simulink model "sedemo_shared_buffer_mgmt"  (Simulink 7.5)
settings: Solver=VariableStepDiscrete  StartTime=0.0  StopTime=10  MaxStep=inf  RelTol=1e-3
undefined symbols (not defined in the file or in its folder): des_subsystemblock, des_subsysteminport, des_subsystemoutport, des_subsystemsupportblock
libraries: simeventstranslate1 x25, simeventssink1 x23, simeventsrouting1 x9, simeventsgates1 x6, simeventsattributes2 x6, simeventsgenerators1 x6, simeventsserver1 x3, simeventsqueue1 x2, simulink x1, simeventsinfo x1
(part 3 of 4)

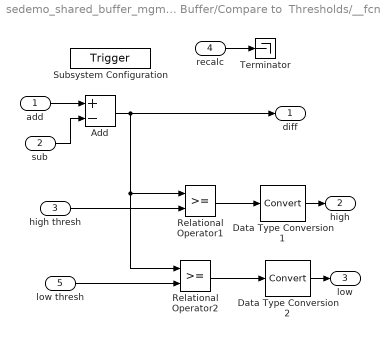
== system sedemo_shared_buffer_mgmt/Receive Buffer/Compare to  Thresholds/__fcn_ss__ ==
  add : Inport  LoadFcn=des_subsysteminport(gcb, 'load');  InitFcn=des_subsysteminport(gcb, 'init');  StartFcn=des_subsysteminport(gcb, 'start');  StopFcn=des_subsysteminport(gcb, 'stop');  OutDataType=sfix(16)  OutScaling=2^0  mask(Discrete Event Inport){PermitSubsystemEvents=on, TypeOfEvent=Change in signal, SignalEdgeOption=Either, SpecifyEventPriority=off, PrioritySubsystemEvent=20}
      mask prompts: PermitSubsystemEvents "Execute subsystem upon signal-based events"; TypeOfEvent "Type of signal-based event:"; SignalEdgeOption "Type of change in signal value:"; SpecifyEventPriority "Resolve simultaneous signal updates according to event priority"; PrioritySubsystemEvent "Event priority:"
      mask help: Input port for a Discrete Event Subsystem block. This block can conditionally execute the subsystem upon signal-based events that meet specified criteria.
      mask init:
      | des_subsystemmask(gcb, 'init','apply')
      settings: CopyFcn=des_subsysteminport(gcb, 'copy');  DeleteFcn=des_subsysteminport(gcb, 'delete');  UndoDeleteFcn=des_subsysteminport(gcb, 'undodelete');  ModelCloseFcn=des_subsysteminport(gcb, 'modelclose');  PreSaveFcn=des_subsysteminport(gcb, 'presave');  NameChangeFcn=des_subsysteminport(gcb, 'namechange');  ParentCloseFcn=des_subsysteminport(gcb, 'parentclose');
      mask Help: helpview(simeventsbhelp);
      mask StyleString: checkbox,popup(Change in signal|Trigger|Sample time hit),popup(Rising|Falling|Either),checkbox,edit
      mask CallbackString: des_subsystemmask(gcb, 'cbPermitSubsystemEvents', 'noapply');|des_subsystemmask(gcb,'cbTypeOfEvent','noapply');||des_subsystemmask(gcb, 'cbSpecifyEventPriority', 'noapply');|
  sub : Inport  LoadFcn=des_subsysteminport(gcb, 'load');  InitFcn=des_subsysteminport(gcb, 'init');  StartFcn=des_subsysteminport(gcb, 'start');  StopFcn=des_subsysteminport(gcb, 'stop');  Port=2  OutDataType=sfix(16)  OutScaling=2^0  mask(Discrete Event Inport){PermitSubsystemEvents=on, TypeOfEvent=Change in signal, SignalEdgeOption=Either, SpecifyEventPriority=on, PrioritySubsystemEvent=20}
      mask prompts: PermitSubsystemEvents "Execute subsystem upon signal-based events"; TypeOfEvent "Type of signal-based event:"; SignalEdgeOption "Type of change in signal value:"; SpecifyEventPriority "Resolve simultaneous signal updates according to event priority"; PrioritySubsystemEvent "Event priority:"
      mask help: Input port for a Discrete Event Subsystem block. This block can conditionally execute the subsystem upon signal-based events that meet specified criteria.
      mask init:
      | des_subsystemmask(gcb, 'init','apply')
      settings: CopyFcn=des_subsysteminport(gcb, 'copy');  DeleteFcn=des_subsysteminport(gcb, 'delete');  UndoDeleteFcn=des_subsysteminport(gcb, 'undodelete');  ModelCloseFcn=des_subsysteminport(gcb, 'modelclose');  PreSaveFcn=des_subsysteminport(gcb, 'presave');  NameChangeFcn=des_subsysteminport(gcb, 'namechange');  ParentCloseFcn=des_subsysteminport(gcb, 'parentclose');
      mask Help: helpview(simeventsbhelp);
      mask StyleString: checkbox,popup(Change in signal|Trigger|Sample time hit),popup(Rising|Falling|Either),checkbox,edit
      mask CallbackString: des_subsystemmask(gcb, 'cbPermitSubsystemEvents', 'noapply');|des_subsystemmask(gcb,'cbTypeOfEvent','noapply');||des_subsystemmask(gcb, 'cbSpecifyEventPriority', 'noapply');|
  high thresh : Inport  LoadFcn=des_subsysteminport(gcb, 'load');  InitFcn=des_subsysteminport(gcb, 'init');  StartFcn=des_subsysteminport(gcb, 'start');  StopFcn=des_subsysteminport(gcb, 'stop');  Port=3  OutDataType=sfix(16)  OutScaling=2^0  mask(Discrete Event Inport){PermitSubsystemEvents=on, TypeOfEvent=Change in signal, SignalEdgeOption=Either, SpecifyEventPriority=off, PrioritySubsystemEvent=20}
      mask prompts: PermitSubsystemEvents "Execute subsystem upon signal-based events"; TypeOfEvent "Type of signal-based event:"; SignalEdgeOption "Type of change in signal value:"; SpecifyEventPriority "Resolve simultaneous signal updates according to event priority"; PrioritySubsystemEvent "Event priority:"
      mask help: Input port for a Discrete Event Subsystem block. This block can conditionally execute the subsystem upon signal-based events that meet specified criteria.
      mask init:
      | des_subsystemmask(gcb, 'init','apply')
      settings: CopyFcn=des_subsysteminport(gcb, 'copy');  DeleteFcn=des_subsysteminport(gcb, 'delete');  UndoDeleteFcn=des_subsysteminport(gcb, 'undodelete');  ModelCloseFcn=des_subsysteminport(gcb, 'modelclose');  PreSaveFcn=des_subsysteminport(gcb, 'presave');  NameChangeFcn=des_subsysteminport(gcb, 'namechange');  ParentCloseFcn=des_subsysteminport(gcb, 'parentclose');
      mask Help: helpview(simeventsbhelp);
      mask StyleString: checkbox,popup(Change in signal|Trigger|Sample time hit),popup(Rising|Falling|Either),checkbox,edit
      mask CallbackString: des_subsystemmask(gcb, 'cbPermitSubsystemEvents', 'noapply');|des_subsystemmask(gcb,'cbTypeOfEvent','noapply');||des_subsystemmask(gcb, 'cbSpecifyEventPriority', 'noapply');|
  recalc : Inport  LoadFcn=des_subsysteminport(gcb, 'load');  InitFcn=des_subsysteminport(gcb, 'init');  StartFcn=des_subsysteminport(gcb, 'start');  StopFcn=des_subsysteminport(gcb, 'stop');  Port=4  OutDataType=sfix(16)  OutScaling=2^0  mask(Discrete Event Inport){PermitSubsystemEvents=on, TypeOfEvent=Change in signal, SignalEdgeOption=Either, SpecifyEventPriority=off, PrioritySubsystemEvent=20}
      mask prompts: PermitSubsystemEvents "Execute subsystem upon signal-based events"; TypeOfEvent "Type of signal-based event:"; SignalEdgeOption "Type of change in signal value:"; SpecifyEventPriority "Resolve simultaneous signal updates according to event priority"; PrioritySubsystemEvent "Event priority:"
      mask help: Input port for a Discrete Event Subsystem block. This block can conditionally execute the subsystem upon signal-based events that meet specified criteria.
      mask init:
      | des_subsystemmask(gcb, 'init','apply')
      settings: CopyFcn=des_subsysteminport(gcb, 'copy');  DeleteFcn=des_subsysteminport(gcb, 'delete');  UndoDeleteFcn=des_subsysteminport(gcb, 'undodelete');  ModelCloseFcn=des_subsysteminport(gcb, 'modelclose');  PreSaveFcn=des_subsysteminport(gcb, 'presave');  NameChangeFcn=des_subsysteminport(gcb, 'namechange');  ParentCloseFcn=des_subsysteminport(gcb, 'parentclose');
      mask Help: helpview(simeventsbhelp);
      mask StyleString: checkbox,popup(Change in signal|Trigger|Sample time hit),popup(Rising|Falling|Either),checkbox,edit
      mask CallbackString: des_subsystemmask(gcb, 'cbPermitSubsystemEvents', 'noapply');|des_subsystemmask(gcb,'cbTypeOfEvent','noapply');||des_subsystemmask(gcb, 'cbSpecifyEventPriority', 'noapply');|
  low thresh : Inport  LoadFcn=des_subsysteminport(gcb, 'load');  InitFcn=des_subsysteminport(gcb, 'init');  StartFcn=des_subsysteminport(gcb, 'start');  StopFcn=des_subsysteminport(gcb, 'stop');  Port=5  OutDataType=sfix(16)  OutScaling=2^0  mask(Discrete Event Inport){PermitSubsystemEvents=on, TypeOfEvent=Change in signal, SignalEdgeOption=Either, SpecifyEventPriority=off, PrioritySubsystemEvent=20}
      mask prompts: PermitSubsystemEvents "Execute subsystem upon signal-based events"; TypeOfEvent "Type of signal-based event:"; SignalEdgeOption "Type of change in signal value:"; SpecifyEventPriority "Resolve simultaneous signal updates according to event priority"; PrioritySubsystemEvent "Event priority:"
      mask help: Input port for a Discrete Event Subsystem block. This block can conditionally execute the subsystem upon signal-based events that meet specified criteria.
      mask init:
      | des_subsystemmask(gcb, 'init','apply')
      settings: CopyFcn=des_subsysteminport(gcb, 'copy');  DeleteFcn=des_subsysteminport(gcb, 'delete');  UndoDeleteFcn=des_subsysteminport(gcb, 'undodelete');  ModelCloseFcn=des_subsysteminport(gcb, 'modelclose');  PreSaveFcn=des_subsysteminport(gcb, 'presave');  NameChangeFcn=des_subsysteminport(gcb, 'namechange');  ParentCloseFcn=des_subsysteminport(gcb, 'parentclose');
      mask Help: helpview(simeventsbhelp);
      mask StyleString: checkbox,popup(Change in signal|Trigger|Sample time hit),popup(Rising|Falling|Either),checkbox,edit
      mask CallbackString: des_subsystemmask(gcb, 'cbPermitSubsystemEvents', 'noapply');|des_subsystemmask(gcb,'cbTypeOfEvent','noapply');||des_subsystemmask(gcb, 'cbSpecifyEventPriority', 'noapply');|
  Subsystem Configuration : TriggerPort  TriggerType=function-call
      settings: CopyFcn=des_subsystemconfigblock(gcb, 'copy');  DeleteFcn=des_subsystemconfigblock(gcb, 'delete');  UndoDeleteFcn=des_subsystemconfigblock(gcb, 'undodelete');
      mask Type: Subsystem Configuration
      mask Description: Configuration for a Discrete Event Subsystem block. Every discrete event subsystem window must contain exactly one copy of this configuration block. Do not delete this block.
      mask Help: helpview(simeventsbhelp);
      mask Display: disp('Do Not Delete');
  Add : Sum  Inputs=+-  OutDataType=sfix(16)  OutScaling=2^-10
  Data Type Conversion1 : DataTypeConversion  OutDataType=sfix(16)  OutScaling=2^0
  Data Type Conversion2 : DataTypeConversion  OutDataType=sfix(16)  OutScaling=2^0
  Relational Operator1 : RelationalOperator  LogicOutDataTypeMode=boolean  OutDataTypeStr=boolean
  Relational Operator2 : RelationalOperator  LogicOutDataTypeMode=boolean  OutDataTypeStr=boolean
  Terminator : Terminator
  diff : Outport  LoadFcn=des_subsystemoutport(gcb, 'load');  InitFcn=des_subsystemoutport(gcb, 'init');  StartFcn=des_subsystemoutport(gcb, 'start');  StopFcn=des_subsystemoutport(gcb, 'stop');  OutDataType=sfix(16)  OutScaling=2^0  mask(Discrete Event Outport){InitOutput=[]}
      mask prompts: InitOutput "Initial output:"
      mask help: Provide an output port for a Discrete Event Subsystem block.
      settings: CopyFcn=des_subsystemoutport(gcb, 'copy');  DeleteFcn=des_subsystemoutport(gcb, 'delete');  UndoDeleteFcn=des_subsystemoutport(gcb, 'undodelete');  ModelCloseFcn=des_subsystemoutport(gcb, 'modelclose');  PreSaveFcn=des_subsystemoutport(gcb, 'presave');  NameChangeFcn=des_subsystemoutport(gcb, 'namechange');  ParentCloseFcn=des_subsystemoutport(gcb, 'parentclose');
      mask Help: helpview(simeventsbhelp);
      mask CallbackString: set_param(gcb,'InitialOutput',get_param(gcb,'InitOutput'));
  high : Outport  LoadFcn=des_subsystemoutport(gcb, 'load');  InitFcn=des_subsystemoutport(gcb, 'init');  StartFcn=des_subsystemoutport(gcb, 'start');  StopFcn=des_subsystemoutport(gcb, 'stop');  Port=2  OutDataType=sfix(16)  OutScaling=2^0  mask(Discrete Event Outport){InitOutput=[]}
      mask prompts: InitOutput "Initial output:"
      mask help: Provide an output port for a Discrete Event Subsystem block.
      settings: CopyFcn=des_subsystemoutport(gcb, 'copy');  DeleteFcn=des_subsystemoutport(gcb, 'delete');  UndoDeleteFcn=des_subsystemoutport(gcb, 'undodelete');  ModelCloseFcn=des_subsystemoutport(gcb, 'modelclose');  PreSaveFcn=des_subsystemoutport(gcb, 'presave');  NameChangeFcn=des_subsystemoutport(gcb, 'namechange');  ParentCloseFcn=des_subsystemoutport(gcb, 'parentclose');
      mask Help: helpview(simeventsbhelp);
      mask CallbackString: set_param(gcb,'InitialOutput',get_param(gcb,'InitOutput'));
  low : Outport  LoadFcn=des_subsystemoutport(gcb, 'load');  InitFcn=des_subsystemoutport(gcb, 'init');  StartFcn=des_subsystemoutport(gcb, 'start');  StopFcn=des_subsystemoutport(gcb, 'stop');  Port=3  OutDataType=sfix(16)  OutScaling=2^0  mask(Discrete Event Outport){InitOutput=[]}
      mask prompts: InitOutput "Initial output:"
      mask help: Provide an output port for a Discrete Event Subsystem block.
      settings: CopyFcn=des_subsystemoutport(gcb, 'copy');  DeleteFcn=des_subsystemoutport(gcb, 'delete');  UndoDeleteFcn=des_subsystemoutport(gcb, 'undodelete');  ModelCloseFcn=des_subsystemoutport(gcb, 'modelclose');  PreSaveFcn=des_subsystemoutport(gcb, 'presave');  NameChangeFcn=des_subsystemoutport(gcb, 'namechange');  ParentCloseFcn=des_subsystemoutport(gcb, 'parentclose');
      mask Help: helpview(simeventsbhelp);
      mask CallbackString: set_param(gcb,'InitialOutput',get_param(gcb,'InitOutput'));
  wires:
  high thresh/1 -> Relational Operator1/2
  add/1 -> Add/1
  sub/1 -> Add/2
  Add/1 -> diff/1, Relational Operator1/1, Relational Operator2/1
  recalc/1 -> Terminator/1
  Data Type Conversion1/1 -> high/1
  Relational Operator1/1 -> Data Type Conversion1/1
  Data Type Conversion2/1 -> low/1
  Relational Operator2/1 -> Data Type Conversion2/1
  low thresh/1 -> Relational Operator2/2

== system sedemo_shared_buffer_mgmt/Receive Buffer/Space Allocated/AAA___ ==

== system sedemo_shared_buffer_mgmt/Receive Buffer/Space Allocated/__fcn_ss__ ==
  add : Inport  LoadFcn=des_subsysteminport(gcb, 'load');  InitFcn=des_subsysteminport(gcb, 'init');  StartFcn=des_subsysteminport(gcb, 'start');  StopFcn=des_subsysteminport(gcb, 'stop');  OutDataType=sfix(16)  OutScaling=2^0  mask(Discrete Event Inport){PermitSubsystemEvents=on, TypeOfEvent=Sample time hit, SignalEdgeOption=Either, SpecifyEventPriority=off, PrioritySubsystemEvent=20}
      mask prompts: PermitSubsystemEvents "Execute subsystem upon signal-based events"; TypeOfEvent "Type of signal-based event:"; SignalEdgeOption "Type of change in signal value:"; SpecifyEventPriority "Resolve simultaneous signal updates according to event priority"; PrioritySubsystemEvent "Event priority:"
      mask help: Input port for a Discrete Event Subsystem block. This block can conditionally execute the subsystem upon signal-based events that meet specified criteria.
      mask init:
      | des_subsystemmask(gcb, 'init','apply')
      settings: CopyFcn=des_subsysteminport(gcb, 'copy');  DeleteFcn=des_subsysteminport(gcb, 'delete');  UndoDeleteFcn=des_subsysteminport(gcb, 'undodelete');  ModelCloseFcn=des_subsysteminport(gcb, 'modelclose');  PreSaveFcn=des_subsysteminport(gcb, 'presave');  NameChangeFcn=des_subsysteminport(gcb, 'namechange');  ParentCloseFcn=des_subsysteminport(gcb, 'parentclose');
      mask Help: helpview(simeventsbhelp);
      mask StyleString: checkbox,popup(Change in signal|Trigger|Sample time hit),popup(Rising|Falling|Either),checkbox,edit
      mask CallbackString: des_subsystemmask(gcb, 'cbPermitSubsystemEvents', 'noapply');|des_subsystemmask(gcb,'cbTypeOfEvent','noapply');||des_subsystemmask(gcb, 'cbSpecifyEventPriority', 'noapply');|
  Subsystem Configuration : TriggerPort  TriggerType=function-call
      settings: CopyFcn=des_subsystemconfigblock(gcb, 'copy');  DeleteFcn=des_subsystemconfigblock(gcb, 'delete');  UndoDeleteFcn=des_subsystemconfigblock(gcb, 'undodelete');
      mask Type: Subsystem Configuration
      mask Description: Configuration for a Discrete Event Subsystem block. Every discrete event subsystem window must contain exactly one copy of this configuration block. Do not delete this block.
      mask Help: helpview(simeventsbhelp);
      mask Display: disp('Do Not Delete');
  Add : Sum  OutDataType=sfix(16)  OutScaling=2^-10
  Unit Delay : UnitDelay  SampleTime=-1
  Acc : Outport  LoadFcn=des_subsystemoutport(gcb, 'load');  InitFcn=des_subsystemoutport(gcb, 'init');  StartFcn=des_subsystemoutport(gcb, 'start');  StopFcn=des_subsystemoutport(gcb, 'stop');  OutDataType=sfix(16)  OutScaling=2^0  mask(Discrete Event Outport){InitOutput=[]}
      mask prompts: InitOutput "Initial output:"
      mask help: Provide an output port for a Discrete Event Subsystem block.
      settings: CopyFcn=des_subsystemoutport(gcb, 'copy');  DeleteFcn=des_subsystemoutport(gcb, 'delete');  UndoDeleteFcn=des_subsystemoutport(gcb, 'undodelete');  ModelCloseFcn=des_subsystemoutport(gcb, 'modelclose');  PreSaveFcn=des_subsystemoutport(gcb, 'presave');  NameChangeFcn=des_subsystemoutport(gcb, 'namechange');  ParentCloseFcn=des_subsystemoutport(gcb, 'parentclose');
      mask Help: helpview(simeventsbhelp);
      mask CallbackString: set_param(gcb,'InitialOutput',get_param(gcb,'InitOutput'));
  wires:
  add/1 -> Add/1
  Unit Delay/1 -> Add/2
  Add/1 -> Unit Delay/1, Acc/1

== system sedemo_shared_buffer_mgmt/Receive Buffer/Space Freed/AAA___ ==

== system sedemo_shared_buffer_mgmt/Receive Buffer/Space Freed/__fcn_ss__ ==
  add : Inport  LoadFcn=des_subsysteminport(gcb, 'load');  InitFcn=des_subsysteminport(gcb, 'init');  StartFcn=des_subsysteminport(gcb, 'start');  StopFcn=des_subsysteminport(gcb, 'stop');  OutDataType=sfix(16)  OutScaling=2^0  mask(Discrete Event Inport){PermitSubsystemEvents=on, TypeOfEvent=Sample time hit, SignalEdgeOption=Either, SpecifyEventPriority=off, PrioritySubsystemEvent=20}
      mask prompts: PermitSubsystemEvents "Execute subsystem upon signal-based events"; TypeOfEvent "Type of signal-based event:"; SignalEdgeOption "Type of change in signal value:"; SpecifyEventPriority "Resolve simultaneous signal updates according to event priority"; PrioritySubsystemEvent "Event priority:"
      mask help: Input port for a Discrete Event Subsystem block. This block can conditionally execute the subsystem upon signal-based events that meet specified criteria.
      mask init:
      | des_subsystemmask(gcb, 'init','apply')
      settings: CopyFcn=des_subsysteminport(gcb, 'copy');  DeleteFcn=des_subsysteminport(gcb, 'delete');  UndoDeleteFcn=des_subsysteminport(gcb, 'undodelete');  ModelCloseFcn=des_subsysteminport(gcb, 'modelclose');  PreSaveFcn=des_subsysteminport(gcb, 'presave');  NameChangeFcn=des_subsysteminport(gcb, 'namechange');  ParentCloseFcn=des_subsysteminport(gcb, 'parentclose');
      mask Help: helpview(simeventsbhelp);
      mask StyleString: checkbox,popup(Change in signal|Trigger|Sample time hit),popup(Rising|Falling|Either),checkbox,edit
      mask CallbackString: des_subsystemmask(gcb, 'cbPermitSubsystemEvents', 'noapply');|des_subsystemmask(gcb,'cbTypeOfEvent','noapply');||des_subsystemmask(gcb, 'cbSpecifyEventPriority', 'noapply');|
  Subsystem Configuration : TriggerPort  TriggerType=function-call
      settings: CopyFcn=des_subsystemconfigblock(gcb, 'copy');  DeleteFcn=des_subsystemconfigblock(gcb, 'delete');  UndoDeleteFcn=des_subsystemconfigblock(gcb, 'undodelete');
      mask Type: Subsystem Configuration
      mask Description: Configuration for a Discrete Event Subsystem block. Every discrete event subsystem window must contain exactly one copy of this configuration block. Do not delete this block.
      mask Help: helpview(simeventsbhelp);
      mask Display: disp('Do Not Delete');
  Add : Sum  OutDataType=sfix(16)  OutScaling=2^-10
  Unit Delay : UnitDelay  SampleTime=-1
  Acc : Outport  LoadFcn=des_subsystemoutport(gcb, 'load');  InitFcn=des_subsystemoutport(gcb, 'init');  StartFcn=des_subsystemoutport(gcb, 'start');  StopFcn=des_subsystemoutport(gcb, 'stop');  OutDataType=sfix(16)  OutScaling=2^0  mask(Discrete Event Outport){InitOutput=[]}
      mask prompts: InitOutput "Initial output:"
      mask help: Provide an output port for a Discrete Event Subsystem block.
      settings: CopyFcn=des_subsystemoutport(gcb, 'copy');  DeleteFcn=des_subsystemoutport(gcb, 'delete');  UndoDeleteFcn=des_subsystemoutport(gcb, 'undodelete');  ModelCloseFcn=des_subsystemoutport(gcb, 'modelclose');  PreSaveFcn=des_subsystemoutport(gcb, 'presave');  NameChangeFcn=des_subsystemoutport(gcb, 'namechange');  ParentCloseFcn=des_subsystemoutport(gcb, 'parentclose');
      mask Help: helpview(simeventsbhelp);
      mask CallbackString: set_param(gcb,'InitialOutput',get_param(gcb,'InitOutput'));
  wires:
  add/1 -> Add/1
  Unit Delay/1 -> Add/2
  Add/1 -> Unit Delay/1, Acc/1

== system sedemo_shared_buffer_mgmt/Rx Priority Throttling/OR/AAA___ ==

== system sedemo_shared_buffer_mgmt/Rx Priority Throttling/OR/__fcn_ss__ ==
  Din : Inport  LoadFcn=des_subsysteminport(gcb, 'load');  InitFcn=des_subsysteminport(gcb, 'init');  StartFcn=des_subsysteminport(gcb, 'start');  StopFcn=des_subsysteminport(gcb, 'stop');  OutDataType=sfix(16)  OutScaling=2^0  mask(Discrete Event Inport){PermitSubsystemEvents=on, TypeOfEvent=Sample time hit, SignalEdgeOption=Rising, SpecifyEventPriority=off, PrioritySubsystemEvent=20}
      mask prompts: PermitSubsystemEvents "Execute subsystem upon signal-based events"; TypeOfEvent "Type of signal-based event:"; SignalEdgeOption "Type of change in signal value:"; SpecifyEventPriority "Resolve simultaneous signal updates according to event priority"; PrioritySubsystemEvent "Event priority:"
      mask help: Input port for a Discrete Event Subsystem block. This block can conditionally execute the subsystem upon signal-based events that meet specified criteria.
      mask init:
      | des_subsystemmask(gcb, 'init','apply')
      settings: CopyFcn=des_subsysteminport(gcb, 'copy');  DeleteFcn=des_subsysteminport(gcb, 'delete');  UndoDeleteFcn=des_subsysteminport(gcb, 'undodelete');  ModelCloseFcn=des_subsysteminport(gcb, 'modelclose');  PreSaveFcn=des_subsysteminport(gcb, 'presave');  NameChangeFcn=des_subsysteminport(gcb, 'namechange');  ParentCloseFcn=des_subsysteminport(gcb, 'parentclose');
      mask Help: helpview(simeventsbhelp);
      mask StyleString: checkbox,popup(Change in signal|Trigger|Sample time hit),popup(Rising|Falling|Either),checkbox,edit
      mask CallbackString: des_subsystemmask(gcb, 'cbPermitSubsystemEvents', 'noapply');|des_subsystemmask(gcb,'cbTypeOfEvent','noapply');||des_subsystemmask(gcb, 'cbSpecifyEventPriority', 'noapply');|
  Din1 : Inport  LoadFcn=des_subsysteminport(gcb, 'load');  InitFcn=des_subsysteminport(gcb, 'init');  StartFcn=des_subsysteminport(gcb, 'start');  StopFcn=des_subsysteminport(gcb, 'stop');  Port=2  OutDataType=sfix(16)  OutScaling=2^0  mask(Discrete Event Inport){PermitSubsystemEvents=on, TypeOfEvent=Sample time hit, SignalEdgeOption=Rising, SpecifyEventPriority=off, PrioritySubsystemEvent=20}
      mask prompts: PermitSubsystemEvents "Execute subsystem upon signal-based events"; TypeOfEvent "Type of signal-based event:"; SignalEdgeOption "Type of change in signal value:"; SpecifyEventPriority "Resolve simultaneous signal updates according to event priority"; PrioritySubsystemEvent "Event priority:"
      mask help: Input port for a Discrete Event Subsystem block. This block can conditionally execute the subsystem upon signal-based events that meet specified criteria.
      mask init:
      | des_subsystemmask(gcb, 'init','apply')
      settings: CopyFcn=des_subsysteminport(gcb, 'copy');  DeleteFcn=des_subsysteminport(gcb, 'delete');  UndoDeleteFcn=des_subsysteminport(gcb, 'undodelete');  ModelCloseFcn=des_subsysteminport(gcb, 'modelclose');  PreSaveFcn=des_subsysteminport(gcb, 'presave');  NameChangeFcn=des_subsysteminport(gcb, 'namechange');  ParentCloseFcn=des_subsysteminport(gcb, 'parentclose');
      mask Help: helpview(simeventsbhelp);
      mask StyleString: checkbox,popup(Change in signal|Trigger|Sample time hit),popup(Rising|Falling|Either),checkbox,edit
      mask CallbackString: des_subsystemmask(gcb, 'cbPermitSubsystemEvents', 'noapply');|des_subsystemmask(gcb,'cbTypeOfEvent','noapply');||des_subsystemmask(gcb, 'cbSpecifyEventPriority', 'noapply');|
  Subsystem Configuration : TriggerPort  TriggerType=function-call
      settings: CopyFcn=des_subsystemconfigblock(gcb, 'copy');  DeleteFcn=des_subsystemconfigblock(gcb, 'delete');  UndoDeleteFcn=des_subsystemconfigblock(gcb, 'undodelete');
      mask Type: Subsystem Configuration
      mask Description: Configuration for a Discrete Event Subsystem block. Every discrete event subsystem window must contain exactly one copy of this configuration block. Do not delete this block.
      mask Help: helpview(simeventsbhelp);
      mask Display: disp('Do Not Delete');
  Logical Operator : Logic  AllPortsSameDT=off  OutDataTypeMode=boolean  OutDataTypeStr=boolean
  Logical Operator1 : Logic  Operator=NOT  AllPortsSameDT=off  OutDataTypeMode=Specify via dialog  LogicDataType=float('double')  OutDataTypeStr=float('double')
  Dout : Outport  LoadFcn=des_subsystemoutport(gcb, 'load');  InitFcn=des_subsystemoutport(gcb, 'init');  StartFcn=des_subsystemoutport(gcb, 'start');  StopFcn=des_subsystemoutport(gcb, 'stop');  OutDataType=sfix(16)  OutScaling=2^0  mask(Discrete Event Outport){InitOutput=[]}
      mask prompts: InitOutput "Initial output:"
      mask help: Provide an output port for a Discrete Event Subsystem block.
      settings: CopyFcn=des_subsystemoutport(gcb, 'copy');  DeleteFcn=des_subsystemoutport(gcb, 'delete');  UndoDeleteFcn=des_subsystemoutport(gcb, 'undodelete');  ModelCloseFcn=des_subsystemoutport(gcb, 'modelclose');  PreSaveFcn=des_subsystemoutport(gcb, 'presave');  NameChangeFcn=des_subsystemoutport(gcb, 'namechange');  ParentCloseFcn=des_subsystemoutport(gcb, 'parentclose');
      mask Help: helpview(simeventsbhelp);
      mask CallbackString: set_param(gcb,'InitialOutput',get_param(gcb,'InitOutput'));
  wires:
  Din/1 -> Logical Operator/1
  Din1/1 -> Logical Operator/2
  Logical Operator/1 -> Logical Operator1/1
  Logical Operator1/1 -> Dout/1

== system sedemo_shared_buffer_mgmt/Rx Priority Throttling/OR1/AAA___ ==

== system sedemo_shared_buffer_mgmt/Rx Priority Throttling/OR1/__fcn_ss__ ==
  Din : Inport  LoadFcn=des_subsysteminport(gcb, 'load');  InitFcn=des_subsysteminport(gcb, 'init');  StartFcn=des_subsysteminport(gcb, 'start');  StopFcn=des_subsysteminport(gcb, 'stop');  OutDataType=sfix(16)  OutScaling=2^0  mask(Discrete Event Inport){PermitSubsystemEvents=on, TypeOfEvent=Sample time hit, SignalEdgeOption=Rising, SpecifyEventPriority=off, PrioritySubsystemEvent=20}
      mask prompts: PermitSubsystemEvents "Execute subsystem upon signal-based events"; TypeOfEvent "Type of signal-based event:"; SignalEdgeOption "Type of change in signal value:"; SpecifyEventPriority "Resolve simultaneous signal updates according to event priority"; PrioritySubsystemEvent "Event priority:"
      mask help: Input port for a Discrete Event Subsystem block. This block can conditionally execute the subsystem upon signal-based events that meet specified criteria.
      mask init:
      | des_subsystemmask(gcb, 'init','apply')
      settings: CopyFcn=des_subsysteminport(gcb, 'copy');  DeleteFcn=des_subsysteminport(gcb, 'delete');  UndoDeleteFcn=des_subsysteminport(gcb, 'undodelete');  ModelCloseFcn=des_subsysteminport(gcb, 'modelclose');  PreSaveFcn=des_subsysteminport(gcb, 'presave');  NameChangeFcn=des_subsysteminport(gcb, 'namechange');  ParentCloseFcn=des_subsysteminport(gcb, 'parentclose');
      mask Help: helpview(simeventsbhelp);
      mask StyleString: checkbox,popup(Change in signal|Trigger|Sample time hit),popup(Rising|Falling|Either),checkbox,edit
      mask CallbackString: des_subsystemmask(gcb, 'cbPermitSubsystemEvents', 'noapply');|des_subsystemmask(gcb,'cbTypeOfEvent','noapply');||des_subsystemmask(gcb, 'cbSpecifyEventPriority', 'noapply');|
  Din1 : Inport  LoadFcn=des_subsysteminport(gcb, 'load');  InitFcn=des_subsysteminport(gcb, 'init');  StartFcn=des_subsysteminport(gcb, 'start');  StopFcn=des_subsysteminport(gcb, 'stop');  Port=2  OutDataType=sfix(16)  OutScaling=2^0  mask(Discrete Event Inport){PermitSubsystemEvents=on, TypeOfEvent=Sample time hit, SignalEdgeOption=Rising, SpecifyEventPriority=off, PrioritySubsystemEvent=20}
      mask prompts: PermitSubsystemEvents "Execute subsystem upon signal-based events"; TypeOfEvent "Type of signal-based event:"; SignalEdgeOption "Type of change in signal value:"; SpecifyEventPriority "Resolve simultaneous signal updates according to event priority"; PrioritySubsystemEvent "Event priority:"
      mask help: Input port for a Discrete Event Subsystem block. This block can conditionally execute the subsystem upon signal-based events that meet specified criteria.
      mask init:
      | des_subsystemmask(gcb, 'init','apply')
      settings: CopyFcn=des_subsysteminport(gcb, 'copy');  DeleteFcn=des_subsysteminport(gcb, 'delete');  UndoDeleteFcn=des_subsysteminport(gcb, 'undodelete');  ModelCloseFcn=des_subsysteminport(gcb, 'modelclose');  PreSaveFcn=des_subsysteminport(gcb, 'presave');  NameChangeFcn=des_subsysteminport(gcb, 'namechange');  ParentCloseFcn=des_subsysteminport(gcb, 'parentclose');
      mask Help: helpview(simeventsbhelp);
      mask StyleString: checkbox,popup(Change in signal|Trigger|Sample time hit),popup(Rising|Falling|Either),checkbox,edit
      mask CallbackString: des_subsystemmask(gcb, 'cbPermitSubsystemEvents', 'noapply');|des_subsystemmask(gcb,'cbTypeOfEvent','noapply');||des_subsystemmask(gcb, 'cbSpecifyEventPriority', 'noapply');|
  Subsystem Configuration : TriggerPort  TriggerType=function-call
      settings: CopyFcn=des_subsystemconfigblock(gcb, 'copy');  DeleteFcn=des_subsystemconfigblock(gcb, 'delete');  UndoDeleteFcn=des_subsystemconfigblock(gcb, 'undodelete');
      mask Type: Subsystem Configuration
      mask Description: Configuration for a Discrete Event Subsystem block. Every discrete event subsystem window must contain exactly one copy of this configuration block. Do not delete this block.
      mask Help: helpview(simeventsbhelp);
      mask Display: disp('Do Not Delete');
  Logical Operator : Logic  AllPortsSameDT=off  OutDataTypeMode=boolean  OutDataTypeStr=boolean
  Logical Operator1 : Logic  Operator=NOT  AllPortsSameDT=off  OutDataTypeMode=Specify via dialog  LogicDataType=float('double')  OutDataTypeStr=float('double')
  Dout : Outport  LoadFcn=des_subsystemoutport(gcb, 'load');  InitFcn=des_subsystemoutport(gcb, 'init');  StartFcn=des_subsystemoutport(gcb, 'start');  StopFcn=des_subsystemoutport(gcb, 'stop');  OutDataType=sfix(16)  OutScaling=2^0  mask(Discrete Event Outport){InitOutput=[]}
      mask prompts: InitOutput "Initial output:"
      mask help: Provide an output port for a Discrete Event Subsystem block.
      settings: CopyFcn=des_subsystemoutport(gcb, 'copy');  DeleteFcn=des_subsystemoutport(gcb, 'delete');  UndoDeleteFcn=des_subsystemoutport(gcb, 'undodelete');  ModelCloseFcn=des_subsystemoutport(gcb, 'modelclose');  PreSaveFcn=des_subsystemoutport(gcb, 'presave');  NameChangeFcn=des_subsystemoutport(gcb, 'namechange');  ParentCloseFcn=des_subsystemoutport(gcb, 'parentclose');
      mask Help: helpview(simeventsbhelp);
      mask CallbackString: set_param(gcb,'InitialOutput',get_param(gcb,'InitOutput'));
  wires:
  Din/1 -> Logical Operator/1
  Din1/1 -> Logical Operator/2
  Logical Operator/1 -> Logical Operator1/1
  Logical Operator1/1 -> Dout/1

== system sedemo_shared_buffer_mgmt/Transmit Buffer/Compare to  Thresholds/AAA___ ==

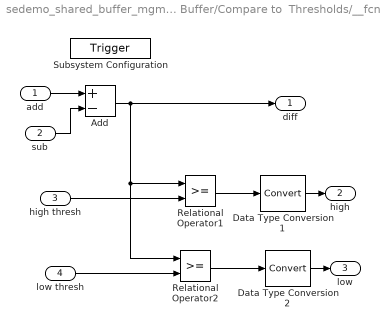
== system sedemo_shared_buffer_mgmt/Transmit Buffer/Compare to  Thresholds/__fcn_ss__ ==
  add : Inport  LoadFcn=des_subsysteminport(gcb, 'load');  InitFcn=des_subsysteminport(gcb, 'init');  StartFcn=des_subsysteminport(gcb, 'start');  StopFcn=des_subsysteminport(gcb, 'stop');  OutDataType=sfix(16)  OutScaling=2^0  mask(Discrete Event Inport){PermitSubsystemEvents=on, TypeOfEvent=Change in signal, SignalEdgeOption=Either, SpecifyEventPriority=off, PrioritySubsystemEvent=20}
      mask prompts: PermitSubsystemEvents "Execute subsystem upon signal-based events"; TypeOfEvent "Type of signal-based event:"; SignalEdgeOption "Type of change in signal value:"; SpecifyEventPriority "Resolve simultaneous signal updates according to event priority"; PrioritySubsystemEvent "Event priority:"
      mask help: Input port for a Discrete Event Subsystem block. This block can conditionally execute the subsystem upon signal-based events that meet specified criteria.
      mask init:
      | des_subsystemmask(gcb, 'init','apply')
      settings: CopyFcn=des_subsysteminport(gcb, 'copy');  DeleteFcn=des_subsysteminport(gcb, 'delete');  UndoDeleteFcn=des_subsysteminport(gcb, 'undodelete');  ModelCloseFcn=des_subsysteminport(gcb, 'modelclose');  PreSaveFcn=des_subsysteminport(gcb, 'presave');  NameChangeFcn=des_subsysteminport(gcb, 'namechange');  ParentCloseFcn=des_subsysteminport(gcb, 'parentclose');
      mask Help: helpview(simeventsbhelp);
      mask StyleString: checkbox,popup(Change in signal|Trigger|Sample time hit),popup(Rising|Falling|Either),checkbox,edit
      mask CallbackString: des_subsystemmask(gcb, 'cbPermitSubsystemEvents', 'noapply');|des_subsystemmask(gcb,'cbTypeOfEvent','noapply');||des_subsystemmask(gcb, 'cbSpecifyEventPriority', 'noapply');|
  sub : Inport  LoadFcn=des_subsysteminport(gcb, 'load');  InitFcn=des_subsysteminport(gcb, 'init');  StartFcn=des_subsysteminport(gcb, 'start');  StopFcn=des_subsysteminport(gcb, 'stop');  Port=2  OutDataType=sfix(16)  OutScaling=2^0  mask(Discrete Event Inport){PermitSubsystemEvents=on, TypeOfEvent=Change in signal, SignalEdgeOption=Either, SpecifyEventPriority=on, PrioritySubsystemEvent=20}
      mask prompts: PermitSubsystemEvents "Execute subsystem upon signal-based events"; TypeOfEvent "Type of signal-based event:"; SignalEdgeOption "Type of change in signal value:"; SpecifyEventPriority "Resolve simultaneous signal updates according to event priority"; PrioritySubsystemEvent "Event priority:"
      mask help: Input port for a Discrete Event Subsystem block. This block can conditionally execute the subsystem upon signal-based events that meet specified criteria.
      mask init:
      | des_subsystemmask(gcb, 'init','apply')
      settings: CopyFcn=des_subsysteminport(gcb, 'copy');  DeleteFcn=des_subsysteminport(gcb, 'delete');  UndoDeleteFcn=des_subsysteminport(gcb, 'undodelete');  ModelCloseFcn=des_subsysteminport(gcb, 'modelclose');  PreSaveFcn=des_subsysteminport(gcb, 'presave');  NameChangeFcn=des_subsysteminport(gcb, 'namechange');  ParentCloseFcn=des_subsysteminport(gcb, 'parentclose');
      mask Help: helpview(simeventsbhelp);
      mask StyleString: checkbox,popup(Change in signal|Trigger|Sample time hit),popup(Rising|Falling|Either),checkbox,edit
      mask CallbackString: des_subsystemmask(gcb, 'cbPermitSubsystemEvents', 'noapply');|des_subsystemmask(gcb,'cbTypeOfEvent','noapply');||des_subsystemmask(gcb, 'cbSpecifyEventPriority', 'noapply');|
  high thresh : Inport  LoadFcn=des_subsysteminport(gcb, 'load');  InitFcn=des_subsysteminport(gcb, 'init');  StartFcn=des_subsysteminport(gcb, 'start');  StopFcn=des_subsysteminport(gcb, 'stop');  Port=3  OutDataType=sfix(16)  OutScaling=2^0  mask(Discrete Event Inport){PermitSubsystemEvents=on, TypeOfEvent=Change in signal, SignalEdgeOption=Either, SpecifyEventPriority=off, PrioritySubsystemEvent=20}
      mask prompts: PermitSubsystemEvents "Execute subsystem upon signal-based events"; TypeOfEvent "Type of signal-based event:"; SignalEdgeOption "Type of change in signal value:"; SpecifyEventPriority "Resolve simultaneous signal updates according to event priority"; PrioritySubsystemEvent "Event priority:"
      mask help: Input port for a Discrete Event Subsystem block. This block can conditionally execute the subsystem upon signal-based events that meet specified criteria.
      mask init:
      | des_subsystemmask(gcb, 'init','apply')
      settings: CopyFcn=des_subsysteminport(gcb, 'copy');  DeleteFcn=des_subsysteminport(gcb, 'delete');  UndoDeleteFcn=des_subsysteminport(gcb, 'undodelete');  ModelCloseFcn=des_subsysteminport(gcb, 'modelclose');  PreSaveFcn=des_subsysteminport(gcb, 'presave');  NameChangeFcn=des_subsysteminport(gcb, 'namechange');  ParentCloseFcn=des_subsysteminport(gcb, 'parentclose');
      mask Help: helpview(simeventsbhelp);
      mask StyleString: checkbox,popup(Change in signal|Trigger|Sample time hit),popup(Rising|Falling|Either),checkbox,edit
      mask CallbackString: des_subsystemmask(gcb, 'cbPermitSubsystemEvents', 'noapply');|des_subsystemmask(gcb,'cbTypeOfEvent','noapply');||des_subsystemmask(gcb, 'cbSpecifyEventPriority', 'noapply');|
  low thresh : Inport  LoadFcn=des_subsysteminport(gcb, 'load');  InitFcn=des_subsysteminport(gcb, 'init');  StartFcn=des_subsysteminport(gcb, 'start');  StopFcn=des_subsysteminport(gcb, 'stop');  Port=4  OutDataType=sfix(16)  OutScaling=2^0  mask(Discrete Event Inport){PermitSubsystemEvents=on, TypeOfEvent=Change in signal, SignalEdgeOption=Either, SpecifyEventPriority=off, PrioritySubsystemEvent=20}
      mask prompts: PermitSubsystemEvents "Execute subsystem upon signal-based events"; TypeOfEvent "Type of signal-based event:"; SignalEdgeOption "Type of change in signal value:"; SpecifyEventPriority "Resolve simultaneous signal updates according to event priority"; PrioritySubsystemEvent "Event priority:"
      mask help: Input port for a Discrete Event Subsystem block. This block can conditionally execute the subsystem upon signal-based events that meet specified criteria.
      mask init:
      | des_subsystemmask(gcb, 'init','apply')
      settings: CopyFcn=des_subsysteminport(gcb, 'copy');  DeleteFcn=des_subsysteminport(gcb, 'delete');  UndoDeleteFcn=des_subsysteminport(gcb, 'undodelete');  ModelCloseFcn=des_subsysteminport(gcb, 'modelclose');  PreSaveFcn=des_subsysteminport(gcb, 'presave');  NameChangeFcn=des_subsysteminport(gcb, 'namechange');  ParentCloseFcn=des_subsysteminport(gcb, 'parentclose');
      mask Help: helpview(simeventsbhelp);
      mask StyleString: checkbox,popup(Change in signal|Trigger|Sample time hit),popup(Rising|Falling|Either),checkbox,edit
      mask CallbackString: des_subsystemmask(gcb, 'cbPermitSubsystemEvents', 'noapply');|des_subsystemmask(gcb,'cbTypeOfEvent','noapply');||des_subsystemmask(gcb, 'cbSpecifyEventPriority', 'noapply');|
  Subsystem Configuration : TriggerPort  TriggerType=function-call
      settings: CopyFcn=des_subsystemconfigblock(gcb, 'copy');  DeleteFcn=des_subsystemconfigblock(gcb, 'delete');  UndoDeleteFcn=des_subsystemconfigblock(gcb, 'undodelete');
      mask Type: Subsystem Configuration
      mask Description: Configuration for a Discrete Event Subsystem block. Every discrete event subsystem window must contain exactly one copy of this configuration block. Do not delete this block.
      mask Help: helpview(simeventsbhelp);
      mask Display: disp('Do Not Delete');
  Add : Sum  Inputs=+-  OutDataType=sfix(16)  OutScaling=2^-10
  Data Type Conversion1 : DataTypeConversion  OutDataType=sfix(16)  OutScaling=2^0
  Data Type Conversion2 : DataTypeConversion  OutDataType=sfix(16)  OutScaling=2^0
  Relational Operator1 : RelationalOperator  LogicOutDataTypeMode=boolean  OutDataTypeStr=boolean
  Relational Operator2 : RelationalOperator  LogicOutDataTypeMode=boolean  OutDataTypeStr=boolean
  diff : Outport  LoadFcn=des_subsystemoutport(gcb, 'load');  InitFcn=des_subsystemoutport(gcb, 'init');  StartFcn=des_subsystemoutport(gcb, 'start');  StopFcn=des_subsystemoutport(gcb, 'stop');  OutDataType=sfix(16)  OutScaling=2^0  mask(Discrete Event Outport){InitOutput=[]}
      mask prompts: InitOutput "Initial output:"
      mask help: Provide an output port for a Discrete Event Subsystem block.
      settings: CopyFcn=des_subsystemoutport(gcb, 'copy');  DeleteFcn=des_subsystemoutport(gcb, 'delete');  UndoDeleteFcn=des_subsystemoutport(gcb, 'undodelete');  ModelCloseFcn=des_subsystemoutport(gcb, 'modelclose');  PreSaveFcn=des_subsystemoutport(gcb, 'presave');  NameChangeFcn=des_subsystemoutport(gcb, 'namechange');  ParentCloseFcn=des_subsystemoutport(gcb, 'parentclose');
      mask Help: helpview(simeventsbhelp);
      mask CallbackString: set_param(gcb,'InitialOutput',get_param(gcb,'InitOutput'));
  high : Outport  LoadFcn=des_subsystemoutport(gcb, 'load');  InitFcn=des_subsystemoutport(gcb, 'init');  StartFcn=des_subsystemoutport(gcb, 'start');  StopFcn=des_subsystemoutport(gcb, 'stop');  Port=2  OutDataType=sfix(16)  OutScaling=2^0  mask(Discrete Event Outport){InitOutput=[]}
      mask prompts: InitOutput "Initial output:"
      mask help: Provide an output port for a Discrete Event Subsystem block.
      settings: CopyFcn=des_subsystemoutport(gcb, 'copy');  DeleteFcn=des_subsystemoutport(gcb, 'delete');  UndoDeleteFcn=des_subsystemoutport(gcb, 'undodelete');  ModelCloseFcn=des_subsystemoutport(gcb, 'modelclose');  PreSaveFcn=des_subsystemoutport(gcb, 'presave');  NameChangeFcn=des_subsystemoutport(gcb, 'namechange');  ParentCloseFcn=des_subsystemoutport(gcb, 'parentclose');
      mask Help: helpview(simeventsbhelp);
      mask CallbackString: set_param(gcb,'InitialOutput',get_param(gcb,'InitOutput'));
  low : Outport  LoadFcn=des_subsystemoutport(gcb, 'load');  InitFcn=des_subsystemoutport(gcb, 'init');  StartFcn=des_subsystemoutport(gcb, 'start');  StopFcn=des_subsystemoutport(gcb, 'stop');  Port=3  OutDataType=sfix(16)  OutScaling=2^0  mask(Discrete Event Outport){InitOutput=[]}
      mask prompts: InitOutput "Initial output:"
      mask help: Provide an output port for a Discrete Event Subsystem block.
      settings: CopyFcn=des_subsystemoutport(gcb, 'copy');  DeleteFcn=des_subsystemoutport(gcb, 'delete');  UndoDeleteFcn=des_subsystemoutport(gcb, 'undodelete');  ModelCloseFcn=des_subsystemoutport(gcb, 'modelclose');  PreSaveFcn=des_subsystemoutport(gcb, 'presave');  NameChangeFcn=des_subsystemoutport(gcb, 'namechange');  ParentCloseFcn=des_subsystemoutport(gcb, 'parentclose');
      mask Help: helpview(simeventsbhelp);
      mask CallbackString: set_param(gcb,'InitialOutput',get_param(gcb,'InitOutput'));
  wires:
  high thresh/1 -> Relational Operator1/2
  add/1 -> Add/1
  sub/1 -> Add/2
  Add/1 -> diff/1, Relational Operator1/1, Relational Operator2/1
  Data Type Conversion1/1 -> high/1
  Relational Operator1/1 -> Data Type Conversion1/1
  Data Type Conversion2/1 -> low/1
  Relational Operator2/1 -> Data Type Conversion2/1
  low thresh/1 -> Relational Operator2/2

== system sedemo_shared_buffer_mgmt/Transmit Buffer/Space Allocated/AAA___ ==

== system sedemo_shared_buffer_mgmt/Transmit Buffer/Space Allocated/__fcn_ss__ ==
  add : Inport  LoadFcn=des_subsysteminport(gcb, 'load');  InitFcn=des_subsysteminport(gcb, 'init');  StartFcn=des_subsysteminport(gcb, 'start');  StopFcn=des_subsysteminport(gcb, 'stop');  OutDataType=sfix(16)  OutScaling=2^0  mask(Discrete Event Inport){PermitSubsystemEvents=on, TypeOfEvent=Sample time hit, SignalEdgeOption=Either, SpecifyEventPriority=off, PrioritySubsystemEvent=20}
      mask prompts: PermitSubsystemEvents "Execute subsystem upon signal-based events"; TypeOfEvent "Type of signal-based event:"; SignalEdgeOption "Type of change in signal value:"; SpecifyEventPriority "Resolve simultaneous signal updates according to event priority"; PrioritySubsystemEvent "Event priority:"
      mask help: Input port for a Discrete Event Subsystem block. This block can conditionally execute the subsystem upon signal-based events that meet specified criteria.
      mask init:
      | des_subsystemmask(gcb, 'init','apply')
      settings: CopyFcn=des_subsysteminport(gcb, 'copy');  DeleteFcn=des_subsysteminport(gcb, 'delete');  UndoDeleteFcn=des_subsysteminport(gcb, 'undodelete');  ModelCloseFcn=des_subsysteminport(gcb, 'modelclose');  PreSaveFcn=des_subsysteminport(gcb, 'presave');  NameChangeFcn=des_subsysteminport(gcb, 'namechange');  ParentCloseFcn=des_subsysteminport(gcb, 'parentclose');
      mask Help: helpview(simeventsbhelp);
      mask StyleString: checkbox,popup(Change in signal|Trigger|Sample time hit),popup(Rising|Falling|Either),checkbox,edit
      mask CallbackString: des_subsystemmask(gcb, 'cbPermitSubsystemEvents', 'noapply');|des_subsystemmask(gcb,'cbTypeOfEvent','noapply');||des_subsystemmask(gcb, 'cbSpecifyEventPriority', 'noapply');|
  Subsystem Configuration : TriggerPort  TriggerType=function-call
      settings: CopyFcn=des_subsystemconfigblock(gcb, 'copy');  DeleteFcn=des_subsystemconfigblock(gcb, 'delete');  UndoDeleteFcn=des_subsystemconfigblock(gcb, 'undodelete');
      mask Type: Subsystem Configuration
      mask Description: Configuration for a Discrete Event Subsystem block. Every discrete event subsystem window must contain exactly one copy of this configuration block. Do not delete this block.
      mask Help: helpview(simeventsbhelp);
      mask Display: disp('Do Not Delete');
  Add : Sum  OutDataType=sfix(16)  OutScaling=2^-10
  Unit Delay : UnitDelay  SampleTime=-1
  Acc : Outport  LoadFcn=des_subsystemoutport(gcb, 'load');  InitFcn=des_subsystemoutport(gcb, 'init');  StartFcn=des_subsystemoutport(gcb, 'start');  StopFcn=des_subsystemoutport(gcb, 'stop');  OutDataType=sfix(16)  OutScaling=2^0  mask(Discrete Event Outport){InitOutput=[]}
      mask prompts: InitOutput "Initial output:"
      mask help: Provide an output port for a Discrete Event Subsystem block.
      settings: CopyFcn=des_subsystemoutport(gcb, 'copy');  DeleteFcn=des_subsystemoutport(gcb, 'delete');  UndoDeleteFcn=des_subsystemoutport(gcb, 'undodelete');  ModelCloseFcn=des_subsystemoutport(gcb, 'modelclose');  PreSaveFcn=des_subsystemoutport(gcb, 'presave');  NameChangeFcn=des_subsystemoutport(gcb, 'namechange');  ParentCloseFcn=des_subsystemoutport(gcb, 'parentclose');
      mask Help: helpview(simeventsbhelp);
      mask CallbackString: set_param(gcb,'InitialOutput',get_param(gcb,'InitOutput'));
  wires:
  add/1 -> Add/1
  Unit Delay/1 -> Add/2
  Add/1 -> Unit Delay/1, Acc/1

== system sedemo_shared_buffer_mgmt/Transmit Buffer/Space Freed/AAA___ ==

== system sedemo_shared_buffer_mgmt/Transmit Buffer/Space Freed/__fcn_ss__ ==
  add : Inport  LoadFcn=des_subsysteminport(gcb, 'load');  InitFcn=des_subsysteminport(gcb, 'init');  StartFcn=des_subsysteminport(gcb, 'start');  StopFcn=des_subsysteminport(gcb, 'stop');  OutDataType=sfix(16)  OutScaling=2^0  mask(Discrete Event Inport){PermitSubsystemEvents=on, TypeOfEvent=Sample time hit, SignalEdgeOption=Either, SpecifyEventPriority=off, PrioritySubsystemEvent=20}
      mask prompts: PermitSubsystemEvents "Execute subsystem upon signal-based events"; TypeOfEvent "Type of signal-based event:"; SignalEdgeOption "Type of change in signal value:"; SpecifyEventPriority "Resolve simultaneous signal updates according to event priority"; PrioritySubsystemEvent "Event priority:"
      mask help: Input port for a Discrete Event Subsystem block. This block can conditionally execute the subsystem upon signal-based events that meet specified criteria.
      mask init:
      | des_subsystemmask(gcb, 'init','apply')
      settings: CopyFcn=des_subsysteminport(gcb, 'copy');  DeleteFcn=des_subsysteminport(gcb, 'delete');  UndoDeleteFcn=des_subsysteminport(gcb, 'undodelete');  ModelCloseFcn=des_subsysteminport(gcb, 'modelclose');  PreSaveFcn=des_subsysteminport(gcb, 'presave');  NameChangeFcn=des_subsysteminport(gcb, 'namechange');  ParentCloseFcn=des_subsysteminport(gcb, 'parentclose');
      mask Help: helpview(simeventsbhelp);
      mask StyleString: checkbox,popup(Change in signal|Trigger|Sample time hit),popup(Rising|Falling|Either),checkbox,edit
      mask CallbackString: des_subsystemmask(gcb, 'cbPermitSubsystemEvents', 'noapply');|des_subsystemmask(gcb,'cbTypeOfEvent','noapply');||des_subsystemmask(gcb, 'cbSpecifyEventPriority', 'noapply');|
  Subsystem Configuration : TriggerPort  TriggerType=function-call
      settings: CopyFcn=des_subsystemconfigblock(gcb, 'copy');  DeleteFcn=des_subsystemconfigblock(gcb, 'delete');  UndoDeleteFcn=des_subsystemconfigblock(gcb, 'undodelete');
      mask Type: Subsystem Configuration
      mask Description: Configuration for a Discrete Event Subsystem block. Every discrete event subsystem window must contain exactly one copy of this configuration block. Do not delete this block.
      mask Help: helpview(simeventsbhelp);
      mask Display: disp('Do Not Delete');
  Add : Sum  OutDataType=sfix(16)  OutScaling=2^-10
  Unit Delay : UnitDelay  SampleTime=-1
  Acc : Outport  LoadFcn=des_subsystemoutport(gcb, 'load');  InitFcn=des_subsystemoutport(gcb, 'init');  StartFcn=des_subsystemoutport(gcb, 'start');  StopFcn=des_subsystemoutport(gcb, 'stop');  OutDataType=sfix(16)  OutScaling=2^0  mask(Discrete Event Outport){InitOutput=[]}
      mask prompts: InitOutput "Initial output:"
      mask help: Provide an output port for a Discrete Event Subsystem block.
      settings: CopyFcn=des_subsystemoutport(gcb, 'copy');  DeleteFcn=des_subsystemoutport(gcb, 'delete');  UndoDeleteFcn=des_subsystemoutport(gcb, 'undodelete');  ModelCloseFcn=des_subsystemoutport(gcb, 'modelclose');  PreSaveFcn=des_subsystemoutport(gcb, 'presave');  NameChangeFcn=des_subsystemoutport(gcb, 'namechange');  ParentCloseFcn=des_subsystemoutport(gcb, 'parentclose');
      mask Help: helpview(simeventsbhelp);
      mask CallbackString: set_param(gcb,'InitialOutput',get_param(gcb,'InitOutput'));
  wires:
  add/1 -> Add/1
  Unit Delay/1 -> Add/2
  Add/1 -> Unit Delay/1, Acc/1

== system sedemo_shared_buffer_mgmt/Tx Priority Throttling/OR/AAA___ ==
